simulink model "quadrotor_backstepping_simulation"  (R2015a)
settings: Solver=ode45  StartTime=0.0  StopTime=15  RelTol=1e-4
values from neighbouring files (symbols this model uses):
  c10 = 1.5    [init_bsgains.m]
  c11 = 2.5    [init_bsgains.m]
  c12 = 1.5    [init_bsgains.m]
  c5 = 13.6263    [init_bsgains.m]    (also in quadrotor_backstepping_controller.m)
  c6 = 13.5392    [init_bsgains.m]    (also in quadrotor_backstepping_controller.m)
  c7 = 2.54    [init_bsgains.m]    (also in quadrotor_backstepping_controller.m)
  c8 = 5.49    [init_bsgains.m]    (also in quadrotor_backstepping_controller.m)
  c9 = 2.5    [init_bsgains.m]
settings Model: Creator=kbmaj  LastModifiedBy=kbmaj

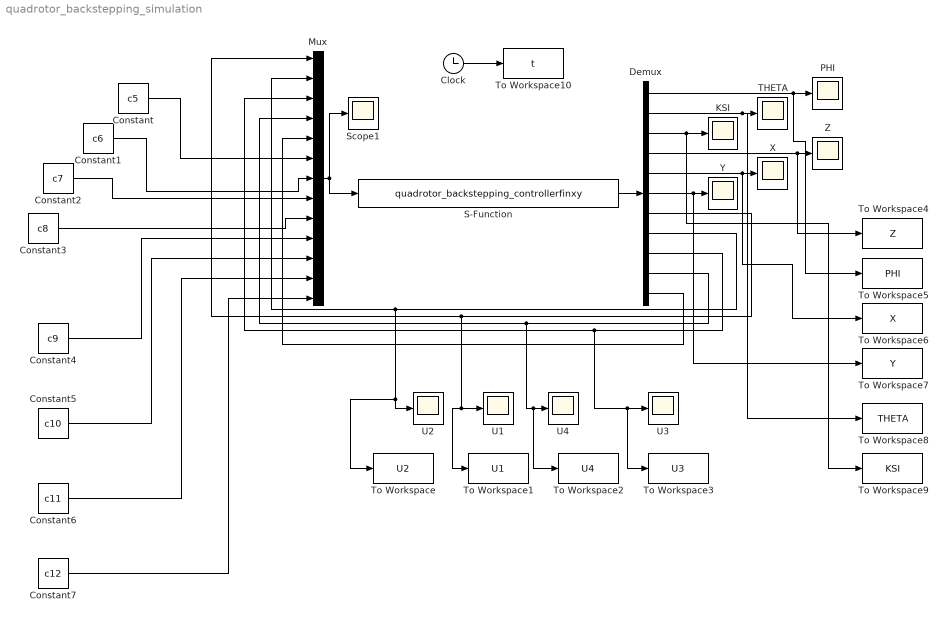
== system quadrotor_backstepping_simulation ==
  Clock : Clock
  Constant : Constant  Value=c5
  Constant1 : Constant  Value=c6
  Constant2 : Constant  Value=c7
  Constant3 : Constant  Value=c8
  Constant4 : Constant  Value=c9
  Constant5 : Constant  Value=c10
  Constant6 : Constant  Value=c11
  Constant7 : Constant  Value=c12
  Demux : Demux  Outputs=11
  KSI : Scope
      settings: YMin=-1359.25  YMax=-1354.25  SaveName=ScopeData4
  Mux : Mux  Inputs=13
  PHI : Scope
      settings: YMin=6.25  YMax=6.55  SaveName=ScopeData2
  S-Function : S-Function  FunctionName=quadrotor_backstepping_controllerfinxy
  Scope1 : Scope
      settings: YMin=-0.5  YMax=6.5
  THETA : Scope
      settings: YMin=19  YMax=21  SaveName=ScopeData3
  To Workspace : ToWorkspace  VariableName=U2  SampleTime=-1
  To Workspace1 : ToWorkspace  VariableName=U1  SampleTime=-1
  To Workspace10 : ToWorkspace  VariableName=t  SampleTime=-1
  To Workspace2 : ToWorkspace  VariableName=U4  SampleTime=-1
  To Workspace3 : ToWorkspace  VariableName=U3  SampleTime=-1
  To Workspace4 : ToWorkspace  VariableName=Z  SampleTime=-1
  To Workspace5 : ToWorkspace  VariableName=PHI  SampleTime=-1
  To Workspace6 : ToWorkspace  VariableName=X  SampleTime=-1
  To Workspace7 : ToWorkspace  VariableName=Y  SampleTime=-1
  To Workspace8 : ToWorkspace  VariableName=THETA  SampleTime=-1
  To Workspace9 : ToWorkspace  VariableName=KSI  SampleTime=-1
  U{1..4} (4 alike) : Scope
      U1 settings: YMin=7.2  YMax=7.5  SaveName=ScopeData9
      U2 settings: YMin=0  YMax=120000  SaveName=ScopeData10
      U3 settings: YMin=0  YMax=120000  SaveName=ScopeData8
      U4 settings: YMin=0  YMax=120000
  X : Scope
      settings: YMin=47450  YMax=47750  SaveName=ScopeData6
  Y : Scope
      settings: YMin=4  YMax=8.5  SaveName=ScopeData7
  Z : Scope
      settings: YMin=9350  YMax=9465  SaveName=ScopeData5
  wires:
  S-Function/1 -> Demux/1
  Mux/1 -> S-Function/1, Scope1/1
  Demux/1 -> To Workspace5/1, PHI/1
  Demux/2 -> To Workspace8/1, THETA/1
  Demux/3 -> To Workspace9/1, KSI/1
  Demux/4 -> To Workspace4/1, Z/1
  Demux/7 -> To Workspace1/1, U1/1, Mux/1
  Demux/9 -> To Workspace3/1, U3/1, Mux/3
  Demux/10 -> To Workspace2/1, U4/1, Mux/4
  Demux/5 -> To Workspace6/1, X/1
  Demux/6 -> To Workspace7/1, Y/1
  Demux/11 -> Mux/5
  Demux/8 -> To Workspace/1, U2/1, Mux/2
  Clock/1 -> To Workspace10/1
  Constant/1 -> Mux/6
  Constant1/1 -> Mux/7
  Constant2/1 -> Mux/8
  Constant3/1 -> Mux/9
  Constant4/1 -> Mux/10
  Constant5/1 -> Mux/11
  Constant6/1 -> Mux/12
  Constant7/1 -> Mux/13
